simulink model "BMS_System_Arch"  (R2024a)
settings: Solver=VariableStepAuto  StartTime=0.0  StopTime=10.0  RelTol=1e-3
model workspace (MAT data in the model file):
  CANBusInterface = Simulink.Bus
  CANBusInterface.Alignment = -1
  CANBusInterface.PreserveElementDimensions = 0
  CANBusInterface.DataScope = 'Auto'
  ChargerInterface = Simulink.Bus
  ChargerInterface.Alignment = -1
  ChargerInterface.PreserveElementDimensions = 0
  ChargerInterface.DataScope = 'Auto'
  DataAcqBus = Simulink.Bus
  DataAcqBus.Alignment = -1
  DataAcqBus.PreserveElementDimensions = 0
  DataAcqBus.DataScope = 'Auto'
  DataCalcBus = Simulink.Bus
  DataCalcBus.Alignment = -1
  DataCalcBus.PreserveElementDimensions = 0
  DataCalcBus.DataScope = 'Auto'
  EstimationBusInterface = Simulink.Bus
  EstimationBusInterface.Alignment = -1
  EstimationBusInterface.PreserveElementDimensions = 0
  EstimationBusInterface.DataScope = 'Auto'
  HMIInterface = Simulink.Bus
  HMIInterface.Alignment = -1
  HMIInterface.PreserveElementDimensions = 0
  HMIInterface.DataScope = 'Auto'
  OperationControl = Simulink.Bus
  OperationControl.Alignment = -1
  OperationControl.PreserveElementDimensions = 0
  OperationControl.DataScope = 'Auto'
  SafetyInterface = Simulink.Bus
  SafetyInterface.Alignment = -1
  SafetyInterface.PreserveElementDimensions = 0
  SafetyInterface.DataScope = 'Auto'
  ThermalInterface = Simulink.Bus
  ThermalInterface.Alignment = -1
  ThermalInterface.PreserveElementDimensions = 0
  ThermalInterface.DataScope = 'Auto'
  UDSInterface = Simulink.Bus
  UDSInterface.Alignment = -1
  UDSInterface.PreserveElementDimensions = 0
  UDSInterface.DataScope = 'Auto'
settings Model: Creator=hirah  LastModifiedBy=hirah

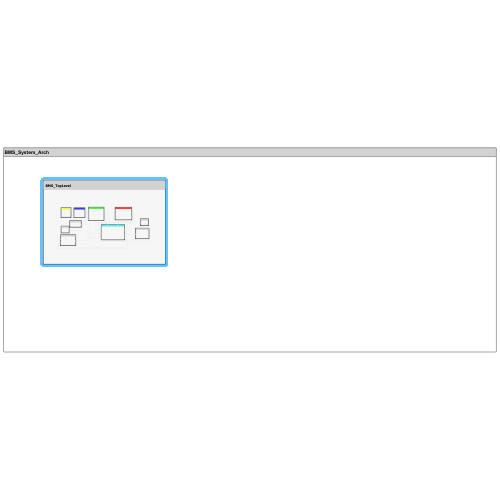
[thumbnail: Simulink's stored preview of the top-level diagram]
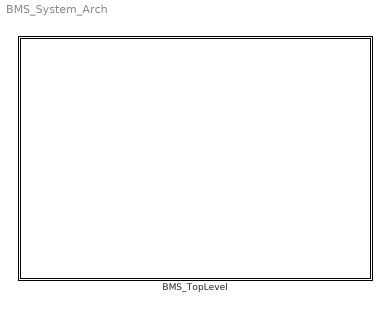
== system BMS_System_Arch ==
  BMS_TopLevel : Subsystem
      settings: PortSchema="{\"entries\":[{\"content\":{\"headerSize\":26,\"margin\":15,\"minimumSpacing\":25,\"sides\":[{\"content\":{},\"type\":\"ConnectorPlacement.EquallySpacedRectSide\",\"uuid\":\"0075fff4-e359-4ca3-82d3-62066e5371b3\"},{\"content\":{\"side\":\"RIGHT\"},\"type\":\"ConnectorPlacement.EquallySpacedRectSide\",\"uuid\":\"0762518f-8ff4-47a0-8585-614cecfccf10\"},{\"content\":{\"side\":\"TOP\"},\"type\":\"ConnectorPlacement.EquallySpacedRectSide\",\"uuid\":\"3af96ac8-a5e6-433b-be31-5dc09c2330cd\"}]},\"type\":\"ConnectorPlacement.EquallySpacedConnector\",\"uuid\":\"5c35ae06-51a0-47e4-81f3-25c096dd406a\"}],\"packageUris\":[\"http://schema.mathworks.com/mf0/Connector/R2020b\"],\"version\":\"1.0\"}"

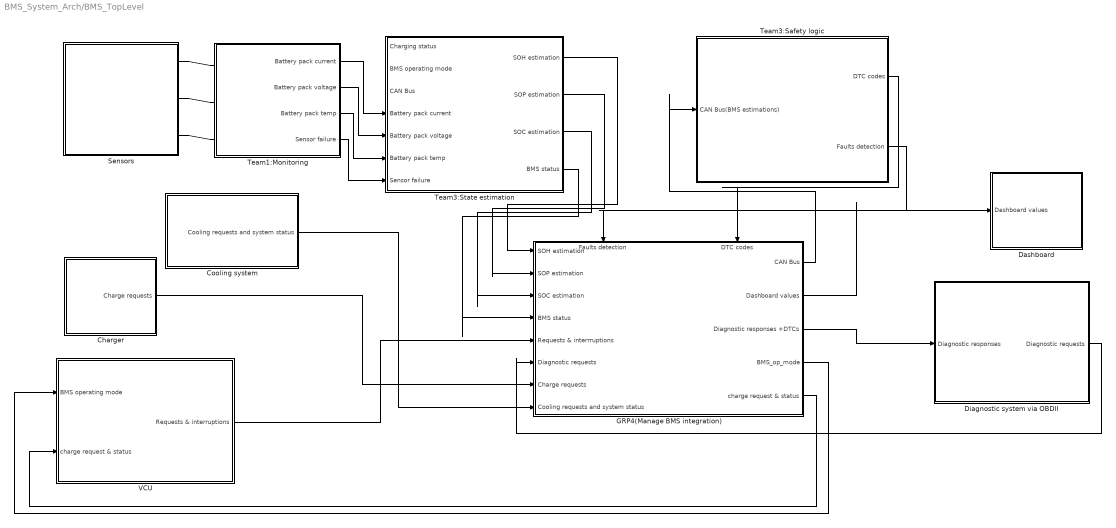
== system BMS_System_Arch/BMS_TopLevel ==
  Charger : Subsystem
      settings: PortSchema="{\"entries\":[{\"content\":{\"headerSize\":26,\"margin\":15,\"minimumSpacing\":25,\"sides\":[{\"content\":{},\"type\":\"ConnectorPlacement.EquallySpacedRectSide\",\"uuid\":\"cd2cdd02-8687-4a8c-9b6e-8ab5b03022cf\"},{\"content\":{\"connectorIds\":[\"Out1\"],\"side\":\"RIGHT\"},\"type\":\"ConnectorPlacement.EquallySpacedRectSide\",\"uuid\":\"c7d3337e-acaa-4958-9ee3-86e02c1b3b1e\"},{\"content\":{\"side\":\"TOP\"},\"type\":\"ConnectorPlacement.EquallySpacedRectSide\",\"uuid\":\"181ed1e6-99e4-4d5e-88b9-0d6c177ff349\"}]},\"type\":\"ConnectorPlacement.EquallySpacedConnector\",\"uuid\":\"35383a89-4be3-49fe-8681-3a2efe2b709c\"}],\"packageUris\":[\"http://schema.mathworks.com/mf0/Connector/R2020b\"],\"version\":\"1.0\"}"
  Cooling system : Subsystem
      settings: PortSchema="{\"entries\":[{\"content\":{\"headerSize\":26,\"margin\":15,\"minimumSpacing\":25,\"sides\":[{\"content\":{},\"type\":\"ConnectorPlacement.EquallySpacedRectSide\",\"uuid\":\"cd2cdd02-8687-4a8c-9b6e-8ab5b03022cf\"},{\"content\":{\"connectorIds\":[\"Out1\"],\"side\":\"RIGHT\"},\"type\":\"ConnectorPlacement.EquallySpacedRectSide\",\"uuid\":\"c7d3337e-acaa-4958-9ee3-86e02c1b3b1e\"},{\"content\":{\"side\":\"TOP\"},\"type\":\"ConnectorPlacement.EquallySpacedRectSide\",\"uuid\":\"181ed1e6-99e4-4d5e-88b9-0d6c177ff349\"}]},\"type\":\"ConnectorPlacement.EquallySpacedConnector\",\"uuid\":\"35383a89-4be3-49fe-8681-3a2efe2b709c\"}],\"packageUris\":[\"http://schema.mathworks.com/mf0/Connector/R2020b\"],\"version\":\"1.0\"}"
  Dashboard : Subsystem
      settings: PortSchema="{\"entries\":[{\"content\":{\"headerSize\":26,\"margin\":15,\"minimumSpacing\":25,\"sides\":[{\"content\":{\"connectorIds\":[\"In1\"]},\"type\":\"ConnectorPlacement.EquallySpacedRectSide\",\"uuid\":\"cd2cdd02-8687-4a8c-9b6e-8ab5b03022cf\"},{\"content\":{\"side\":\"RIGHT\"},\"type\":\"ConnectorPlacement.EquallySpacedRectSide\",\"uuid\":\"c7d3337e-acaa-4958-9ee3-86e02c1b3b1e\"},{\"content\":{\"side\":\"TOP\"},\"type\":\"ConnectorPlacement.EquallySpacedRectSide\",\"uuid\":\"181ed1e6-99e4-4d5e-88b9-0d6c177ff349\"}]},\"type\":\"ConnectorPlacement.EquallySpacedConnector\",\"uuid\":\"35383a89-4be3-49fe-8681-3a2efe2b709c\"}],\"packageUris\":[\"http://schema.mathworks.com/mf0/Connector/R2020b\"],\"version\":\"1.0\"}"
  Diagnostic system via OBDII : Subsystem
      settings: PortSchema="{\"entries\":[{\"content\":{\"headerSize\":26,\"margin\":15,\"minimumSpacing\":25,\"sides\":[{\"content\":{\"connectorIds\":[\"In1\"]},\"type\":\"ConnectorPlacement.EquallySpacedRectSide\",\"uuid\":\"cd2cdd02-8687-4a8c-9b6e-8ab5b03022cf\"},{\"content\":{\"connectorIds\":[\"Out1\"],\"side\":\"RIGHT\"},\"type\":\"ConnectorPlacement.EquallySpacedRectSide\",\"uuid\":\"c7d3337e-acaa-4958-9ee3-86e02c1b3b1e\"},{\"content\":{\"side\":\"TOP\"},\"type\":\"ConnectorPlacement.EquallySpacedRectSide\",\"uuid\":\"181ed1e6-99e4-4d5e-88b9-0d6c177ff349\"}]},\"type\":\"ConnectorPlacement.EquallySpacedConnector\",\"uuid\":\"35383a89-4be3-49fe-8681-3a2efe2b709c\"}],\"packageUris\":[\"http://schema.mathworks.com/mf0/Connector/R2020b\"],\"version\":\"1.0\"}"
  GRP4(Manage BMS integration) : Subsystem
      settings: PortSchema="{\"entries\":[{\"content\":{\"headerSize\":26,\"margin\":15,\"minimumSpacing\":25,\"sides\":[{\"content\":{\"connectorIds\":[\"In3\",\"In4\",\"In8\",\"In9\",\"In10\",\"In5\",\"In6\",\"In7\"]},\"type\":\"ConnectorPlacement.EquallySpacedRectSide\",\"uuid\":\"faff89d9-e9e4-4b6f-9f42-f9315910e0de\"},{\"content\":{\"connectorIds\":[\"Out1\",\"Out2\",\"Out3\",\"Out4\",\"Out5\"],\"side\":\"RIGHT\"},\"type\":\"ConnectorPlacement.EquallySpacedRectSide\",\"uuid\":\"9773bad6-87c4-4101-99c1-1d204d4e17cb\"},{\"content\":{\"connectorIds\":[\"In1\",\"In2\"],\"side\":\"TOP\"},\"type\":\"ConnectorPlacement.EquallySpacedRectSide\",\"uuid\":\"573ffa45-035d-496a-acbc-febfae678741\"}]},\"type\":\"ConnectorPlacement.EquallySpacedConnector\",\"uuid\":\"e66d261f-d4c2-4899-bd49-de4415fbe12f\"}],\"packageUris\":[\"http://schema.mathworks.com/mf0/Connector/R2020b\"],\"version\":\"1.0\"}"
  Sensors : Subsystem
      settings: PortSchema="{\"entries\":[{\"content\":{\"headerSize\":26,\"margin\":15,\"minimumSpacing\":25,\"sides\":[{\"content\":{},\"type\":\"ConnectorPlacement.EquallySpacedRectSide\",\"uuid\":\"faff89d9-e9e4-4b6f-9f42-f9315910e0de\"},{\"content\":{\"connectorIds\":[\"RConn1\",\"RConn2\",\"RConn3\"],\"side\":\"RIGHT\"},\"type\":\"ConnectorPlacement.EquallySpacedRectSide\",\"uuid\":\"9773bad6-87c4-4101-99c1-1d204d4e17cb\"},{\"content\":{\"side\":\"TOP\"},\"type\":\"ConnectorPlacement.EquallySpacedRectSide\",\"uuid\":\"573ffa45-035d-496a-acbc-febfae678741\"}]},\"type\":\"ConnectorPlacement.EquallySpacedConnector\",\"uuid\":\"e66d261f-d4c2-4899-bd49-de4415fbe12f\"}],\"packageUris\":[\"http://schema.mathworks.com/mf0/Connector/R2020b\"],\"version\":\"1.0\"}"
  Team1:Monitoring : Subsystem
      settings: PortSchema="{\"entries\":[{\"content\":{\"headerSize\":26,\"margin\":15,\"minimumSpacing\":25,\"sides\":[{\"content\":{\"connectorIds\":[\"LConn1\",\"LConn2\",\"LConn3\"]},\"type\":\"ConnectorPlacement.EquallySpacedRectSide\",\"uuid\":\"cd2cdd02-8687-4a8c-9b6e-8ab5b03022cf\"},{\"content\":{\"connectorIds\":[\"Out1\",\"Out2\",\"Out3\",\"Out4\"],\"side\":\"RIGHT\"},\"type\":\"ConnectorPlacement.EquallySpacedRectSide\",\"uuid\":\"c7d3337e-acaa-4958-9ee3-86e02c1b3b1e\"},{\"content\":{\"side\":\"TOP\"},\"type\":\"ConnectorPlacement.EquallySpacedRectSide\",\"uuid\":\"181ed1e6-99e4-4d5e-88b9-0d6c177ff349\"}]},\"type\":\"ConnectorPlacement.EquallySpacedConnector\",\"uuid\":\"35383a89-4be3-49fe-8681-3a2efe2b709c\"}],\"packageUris\":[\"http://schema.mathworks.com/mf0/Connector/R2020b\"],\"version\":\"1.0\"}"
  Team3:Safety logic : Subsystem
      settings: PortSchema="{\"entries\":[{\"content\":{\"headerSize\":26,\"margin\":15,\"minimumSpacing\":25,\"sides\":[{\"content\":{\"connectorIds\":[\"In1\"]},\"type\":\"ConnectorPlacement.EquallySpacedRectSide\",\"uuid\":\"cd2cdd02-8687-4a8c-9b6e-8ab5b03022cf\"},{\"content\":{\"connectorIds\":[\"Out1\",\"Out2\"],\"side\":\"RIGHT\"},\"type\":\"ConnectorPlacement.EquallySpacedRectSide\",\"uuid\":\"c7d3337e-acaa-4958-9ee3-86e02c1b3b1e\"},{\"content\":{\"side\":\"TOP\"},\"type\":\"ConnectorPlacement.EquallySpacedRectSide\",\"uuid\":\"181ed1e6-99e4-4d5e-88b9-0d6c177ff349\"}]},\"type\":\"ConnectorPlacement.EquallySpacedConnector\",\"uuid\":\"35383a89-4be3-49fe-8681-3a2efe2b709c\"}],\"packageUris\":[\"http://schema.mathworks.com/mf0/Connector/R2020b\"],\"version\":\"1.0\"}"
  Team3:State estimation : Subsystem
      settings: PortSchema="{\"entries\":[{\"content\":{\"headerSize\":26,\"margin\":15,\"minimumSpacing\":25,\"sides\":[{\"content\":{\"connectorIds\":[\"In1\",\"In2\",\"In3\",\"In4\",\"In5\",\"In6\",\"In7\"]},\"type\":\"ConnectorPlacement.EquallySpacedRectSide\",\"uuid\":\"faff89d9-e9e4-4b6f-9f42-f9315910e0de\"},{\"content\":{\"connectorIds\":[\"Out1\",\"Out2\",\"Out3\",\"Out4\"],\"side\":\"RIGHT\"},\"type\":\"ConnectorPlacement.EquallySpacedRectSide\",\"uuid\":\"9773bad6-87c4-4101-99c1-1d204d4e17cb\"},{\"content\":{\"side\":\"TOP\"},\"type\":\"ConnectorPlacement.EquallySpacedRectSide\",\"uuid\":\"573ffa45-035d-496a-acbc-febfae678741\"}]},\"type\":\"ConnectorPlacement.EquallySpacedConnector\",\"uuid\":\"e66d261f-d4c2-4899-bd49-de4415fbe12f\"}],\"packageUris\":[\"http://schema.mathworks.com/mf0/Connector/R2020b\"],\"version\":\"1.0\"}"
  VCU : Subsystem
      settings: PortSchema="{\"entries\":[{\"content\":{\"headerSize\":26,\"margin\":15,\"minimumSpacing\":25,\"sides\":[{\"content\":{\"connectorIds\":[\"In1\",\"In2\"]},\"type\":\"ConnectorPlacement.EquallySpacedRectSide\",\"uuid\":\"cd2cdd02-8687-4a8c-9b6e-8ab5b03022cf\"},{\"content\":{\"connectorIds\":[\"Out1\"],\"side\":\"RIGHT\"},\"type\":\"ConnectorPlacement.EquallySpacedRectSide\",\"uuid\":\"c7d3337e-acaa-4958-9ee3-86e02c1b3b1e\"},{\"content\":{\"side\":\"TOP\"},\"type\":\"ConnectorPlacement.EquallySpacedRectSide\",\"uuid\":\"181ed1e6-99e4-4d5e-88b9-0d6c177ff349\"}]},\"type\":\"ConnectorPlacement.EquallySpacedConnector\",\"uuid\":\"35383a89-4be3-49fe-8681-3a2efe2b709c\"}],\"packageUris\":[\"http://schema.mathworks.com/mf0/Connector/R2020b\"],\"version\":\"1.0\"}"
  wires:
  Team1:Monitoring/2(Battery pack voltage) -> Team3:State estimation/5(Battery pack voltage)
  Team1:Monitoring/1(Battery pack current) -> Team3:State estimation/4(Battery pack current)
  Team1:Monitoring/3(Battery pack temp) -> Team3:State estimation/6(Battery pack temp)
  Team1:Monitoring/4(Sensor failure) -> Team3:State estimation/7(Sensor failure)
  Team3:State estimation/1(SOH estimation) -> GRP4(Manage BMS integration)/3(SOH estimation)
  Team3:State estimation/2(SOP estimation) -> GRP4(Manage BMS integration)/4(SOP estimation)
  Team3:State estimation/3(SOC estimation) -> GRP4(Manage BMS integration)/8(SOC estimation)
  Team3:State estimation/4(BMS status) -> GRP4(Manage BMS integration)/9(BMS status)
  VCU/1(Requests & interruptions) -> GRP4(Manage BMS integration)/10(Requests & interrruptions)
  GRP4(Manage BMS integration)/1(CAN Bus) -> Team3:Safety logic/1(CAN Bus(BMS estimations))
  Team3:Safety logic/2(Faults detection) -> GRP4(Manage BMS integration)/1(Faults detection)
  Team3:Safety logic/1(DTC codes) -> GRP4(Manage BMS integration)/2(DTC codes)
  GRP4(Manage BMS integration)/4(BMS_op_mode) -> VCU/1(BMS operating mode)
  GRP4(Manage BMS integration)/3(Diagnostic responses +DTCs) -> Diagnostic system via OBDII/1(Diagnostic responses)
  Diagnostic system via OBDII/1(Diagnostic requests) -> GRP4(Manage BMS integration)/5(Diagnostic requests)
  GRP4(Manage BMS integration)/2(Dashboard values) -> Dashboard/1(Dashboard values)
  GRP4(Manage BMS integration)/5(charge request & status) -> VCU/2(charge request & status)
  Charger/1(Charge requests) -> GRP4(Manage BMS integration)/6(Charge requests)
  Cooling system/1(Cooling requests and system status) -> GRP4(Manage BMS integration)/7(Cooling requests and system status)
  connections:
  Sensors/RConn2 -- Team1:Monitoring/LConn2
  Sensors/RConn1 -- Team1:Monitoring/LConn1
  Sensors/RConn3 -- Team1:Monitoring/LConn3

== system BMS_System_Arch/BMS_TopLevel/Charger ==
  Bus Element Out1 : Outport  PortName=Charge requests

== system BMS_System_Arch/BMS_TopLevel/Cooling system ==
  Bus Element Out1 : Outport  PortName=Cooling requests and system status

== system BMS_System_Arch/BMS_TopLevel/Dashboard ==
  Bus Element In1 : Inport  PortName=Dashboard values

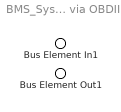
== system BMS_System_Arch/BMS_TopLevel/Diagnostic system via OBDII ==
  Bus Element In1 : Inport  PortName=Diagnostic responses
  Bus Element Out1 : Outport  PortName=Diagnostic requests

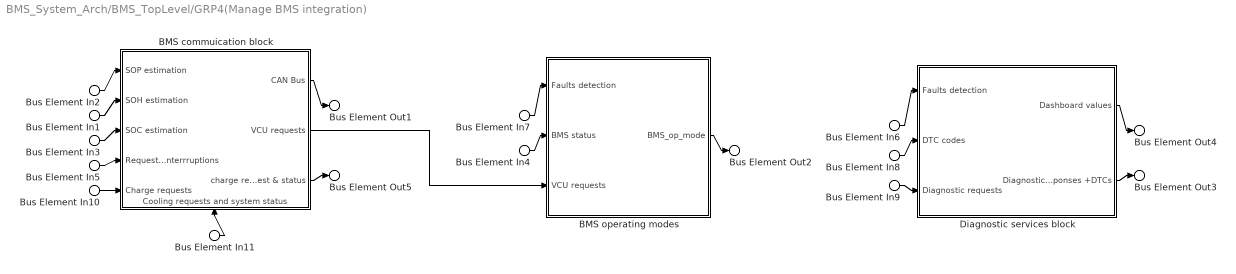
== system BMS_System_Arch/BMS_TopLevel/GRP4(Manage BMS integration) ==
  Bus Element In6 : Inport  PortName=Faults detection
  Bus Element In7 : Inport  PortName=Faults detection
  Bus Element In8 : Inport  Port=2  PortName=DTC codes
  Bus Element In1 : Inport  Port=3  PortName=SOH estimation
  Bus Element In2 : Inport  Port=4  PortName=SOP estimation
  Bus Element In9 : Inport  Port=5  PortName=Diagnostic requests
  Bus Element In10 : Inport  Port=6  PortName=Charge requests
  Bus Element In11 : Inport  Port=7  PortName=Cooling requests and system status
  Bus Element In3 : Inport  Port=8  PortName=SOC estimation
  Bus Element In4 : Inport  Port=9  PortName=BMS status
  Bus Element In5 : Inport  Port=10  PortName=Requests & interrruptions
  BMS commuication block : Subsystem
      settings: PortSchema="{\"entries\":[{\"content\":{\"headerSize\":26,\"margin\":15,\"minimumSpacing\":25,\"sides\":[{\"content\":{\"connectorIds\":[\"In2\",\"In3\",\"In4\",\"In5\",\"In6\"]},\"type\":\"ConnectorPlacement.EquallySpacedRectSide\",\"uuid\":\"04ec415f-b4bd-4017-972b-9e85e691a4fa\"},{\"content\":{\"connectorIds\":[\"Out1\",\"Out2\",\"Out3\"],\"side\":\"RIGHT\"},\"type\":\"ConnectorPlacement.EquallySpacedRectSide\",\"uuid\":\"35151384-2339-42ef-bb6e-a180feceabd8\"},{\"content\":{\"side\":\"TOP\"},\"type\":\"ConnectorPlacement.EquallySpacedRectSide\",\"uuid\":\"c25567f8-acdc-4fac-aea5-0e07a58d33ff\"},{\"content\":{\"connectorIds\":[\"In1\"],\"side\":\"BOTTOM\"},\"type\":\"ConnectorPlacement.EquallySpacedRectSide\",\"uuid\":\"03d92b78-152a-4a99-a80a-d3186856140b\"}]},\"type\":\"ConnectorPlacement.EquallySpacedConnector\",\"uuid\":\"6bdc95ed-225b-47c7-9236-872fc0620aae\"}],\"packageUris\":[\"http://schema.mathworks.com/mf0/Connector/R2020b\"],\"version\":\"1.0\"}"
  BMS operating modes : Subsystem
      settings: PortSchema="{\"entries\":[{\"content\":{\"headerSize\":26,\"margin\":15,\"minimumSpacing\":25,\"sides\":[{\"content\":{\"connectorIds\":[\"In1\",\"In2\",\"In3\"]},\"type\":\"ConnectorPlacement.EquallySpacedRectSide\",\"uuid\":\"faff89d9-e9e4-4b6f-9f42-f9315910e0de\"},{\"content\":{\"connectorIds\":[\"Out1\"],\"side\":\"RIGHT\"},\"type\":\"ConnectorPlacement.EquallySpacedRectSide\",\"uuid\":\"9773bad6-87c4-4101-99c1-1d204d4e17cb\"},{\"content\":{\"side\":\"TOP\"},\"type\":\"ConnectorPlacement.EquallySpacedRectSide\",\"uuid\":\"573ffa45-035d-496a-acbc-febfae678741\"}]},\"type\":\"ConnectorPlacement.EquallySpacedConnector\",\"uuid\":\"e66d261f-d4c2-4899-bd49-de4415fbe12f\"}],\"packageUris\":[\"http://schema.mathworks.com/mf0/Connector/R2020b\"],\"version\":\"1.0\"}"
  Diagnostic services block : Subsystem
      settings: PortSchema="{\"entries\":[{\"content\":{\"headerSize\":26,\"margin\":15,\"minimumSpacing\":25,\"sides\":[{\"content\":{\"connectorIds\":[\"In1\",\"In2\",\"In3\"]},\"type\":\"ConnectorPlacement.EquallySpacedRectSide\",\"uuid\":\"04ec415f-b4bd-4017-972b-9e85e691a4fa\"},{\"content\":{\"connectorIds\":[\"Out1\",\"Out2\"],\"side\":\"RIGHT\"},\"type\":\"ConnectorPlacement.EquallySpacedRectSide\",\"uuid\":\"35151384-2339-42ef-bb6e-a180feceabd8\"},{\"content\":{\"side\":\"TOP\"},\"type\":\"ConnectorPlacement.EquallySpacedRectSide\",\"uuid\":\"c25567f8-acdc-4fac-aea5-0e07a58d33ff\"}]},\"type\":\"ConnectorPlacement.EquallySpacedConnector\",\"uuid\":\"6bdc95ed-225b-47c7-9236-872fc0620aae\"}],\"packageUris\":[\"http://schema.mathworks.com/mf0/Connector/R2020b\"],\"version\":\"1.0\"}"
  Bus Element Out1 : Outport  PortName=CAN Bus
  Bus Element Out4 : Outport  Port=2  PortName=Dashboard values
  Bus Element Out3 : Outport  Port=3  PortName=Diagnostic responses +DTCs
  Bus Element Out2 : Outport  Port=4  PortName=BMS_op_mode
  Bus Element Out5 : Outport  Port=5  PortName=charge request & status
  wires:
  Diagnostic services block/1(Dashboard values) -> Bus Element Out4/1
  Diagnostic services block/2(Diagnostic responses +DTCs) -> Bus Element Out3/1
  BMS commuication block/1(CAN Bus) -> Bus Element Out1/1
  Bus Element In8/1 -> Diagnostic services block/2(DTC codes)
  Bus Element In6/1 -> Diagnostic services block/1(Faults detection)
  Bus Element In1/1 -> BMS commuication block/3(SOH estimation)
  Bus Element In2/1 -> BMS commuication block/2(SOP estimation)
  Bus Element In3/1 -> BMS commuication block/4(SOC estimation)
  Bus Element In4/1 -> BMS operating modes/2(BMS status)
  Bus Element In5/1 -> BMS commuication block/5(Requests & interrruptions)
  BMS commuication block/2(VCU requests) -> BMS operating modes/3(VCU requests)
  Bus Element In9/1 -> Diagnostic services block/3(Diagnostic requests)
  Bus Element In10/1 -> BMS commuication block/6(Charge requests)
  Bus Element In11/1 -> BMS commuication block/1(Cooling requests and system status)
  BMS operating modes/1(BMS_op_mode) -> Bus Element Out2/1
  BMS commuication block/3(charge request & status) -> Bus Element Out5/1
  Bus Element In7/1 -> BMS operating modes/1(Faults detection)

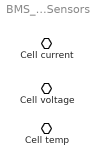
== system BMS_System_Arch/BMS_TopLevel/Sensors ==
  Cell current : PMIOPort  Side=Right
  Cell voltage : PMIOPort  Port=2  Side=Right
  Cell temp : PMIOPort  Port=3  Side=Right

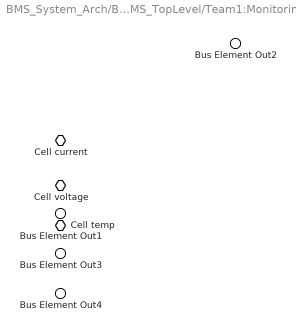
== system BMS_System_Arch/BMS_TopLevel/Team1:Monitoring ==
  Cell current : PMIOPort  Side=Left  ConnectionType=Connection: foundation.electrical.eight_phase
  Cell voltage : PMIOPort  Port=2  Side=Left
  Cell temp : PMIOPort  Port=3  Side=Left
  Bus Element Out2 : Outport  PortName=Battery pack current
  Bus Element Out1 : Outport  Port=2  PortName=Battery pack voltage
  Bus Element Out3 : Outport  Port=3  PortName=Battery pack temp
  Bus Element Out4 : Outport  Port=4  PortName=Sensor failure

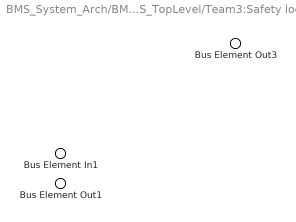
== system BMS_System_Arch/BMS_TopLevel/Team3:Safety logic ==
  Bus Element In1 : Inport  PortName=CAN Bus(BMS estimations)
  Bus Element Out3 : Outport  PortName=DTC codes
  Bus Element Out1 : Outport  Port=2  PortName=Faults detection

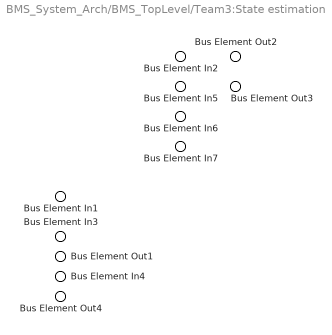
== system BMS_System_Arch/BMS_TopLevel/Team3:State estimation ==
  Bus Element In7 : Inport  PortName=Charging status
  Bus Element In6 : Inport  Port=2  PortName=BMS operating mode
  Bus Element In5 : Inport  Port=3  PortName=CAN Bus
  Bus Element In2 : Inport  Port=4  PortName=Battery pack current
  Bus Element In1 : Inport  Port=5  PortName=Battery pack voltage
  Bus Element In3 : Inport  Port=6  PortName=Battery pack temp
  Bus Element In4 : Inport  Port=7  PortName=Sensor failure
  Bus Element Out2 : Outport  PortName=SOH estimation
  Bus Element Out3 : Outport  Port=2  PortName=SOP estimation
  Bus Element Out1 : Outport  Port=3  PortName=SOC estimation
  Bus Element Out4 : Outport  Port=4  PortName=BMS status

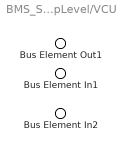
== system BMS_System_Arch/BMS_TopLevel/VCU ==
  Bus Element In1 : Inport  PortName=BMS operating mode
  Bus Element In2 : Inport  Port=2  PortName=charge request & status
  Bus Element Out1 : Outport  PortName=Requests & interruptions

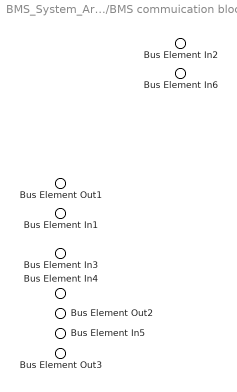
== system BMS_System_Arch/BMS_TopLevel/GRP4(Manage BMS integration)/BMS commuication block ==
  Bus Element In6 : Inport  PortName=Cooling requests and system status
  Bus Element In2 : Inport  Port=2  PortName=SOP estimation
  Bus Element In1 : Inport  Port=3  PortName=SOH estimation
  Bus Element In3 : Inport  Port=4  PortName=SOC estimation
  Bus Element In4 : Inport  Port=5  PortName=Requests & interrruptions
  Bus Element In5 : Inport  Port=6  PortName=Charge requests
  Bus Element Out1 : Outport  PortName=CAN Bus
  Bus Element Out2 : Outport  Port=2  PortName=VCU requests
  Bus Element Out3 : Outport  Port=3  PortName=charge request & status

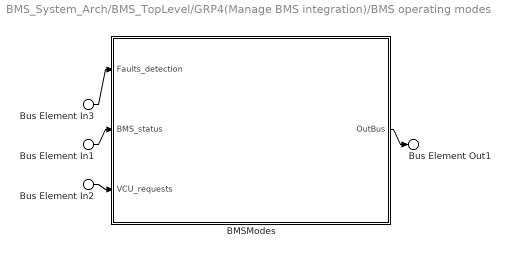
== system BMS_System_Arch/BMS_TopLevel/GRP4(Manage BMS integration)/BMS operating modes ==
  Bus Element In3 : Inport  PortName=Faults detection
  Bus Element In1 : Inport  Port=2  PortName=BMS status
  Bus Element In2 : Inport  Port=3  PortName=VCU requests
  BMSModes : Stateflow chart  TreatAsAtomicUnit=on
      settings: PortSchema="{\"entries\":[{\"content\":{\"headerSize\":26,\"margin\":15,\"minimumSpacing\":25,\"sides\":[{\"content\":{\"connectorIds\":[\"In1\",\"In2\",\"In3\"]},\"type\":\"ConnectorPlacement.EquallySpacedRectSide\",\"uuid\":\"04ec415f-b4bd-4017-972b-9e85e691a4fa\"},{\"content\":{\"connectorIds\":[\"Out1\"],\"side\":\"RIGHT\"},\"type\":\"ConnectorPlacement.EquallySpacedRectSide\",\"uuid\":\"35151384-2339-42ef-bb6e-a180feceabd8\"},{\"content\":{\"side\":\"TOP\"},\"type\":\"ConnectorPlacement.EquallySpacedRectSide\",\"uuid\":\"c25567f8-acdc-4fac-aea5-0e07a58d33ff\"}]},\"type\":\"ConnectorPlacement.EquallySpacedConnector\",\"uuid\":\"6bdc95ed-225b-47c7-9236-872fc0620aae\"}],\"packageUris\":[\"http://schema.mathworks.com/mf0/Connector/R2020b\"],\"version\":\"1.0\"}"
  Bus Element Out1 : Outport  PortName=BMS_op_mode
  wires:
  Bus Element In1/1 -> BMSModes/2(BMS_status)
  Bus Element In2/1 -> BMSModes/3(VCU_requests)
  Bus Element In3/1 -> BMSModes/1(Faults_detection)
  BMSModes/1(OutBus) -> Bus Element Out1/1

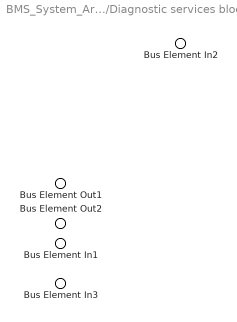
== system BMS_System_Arch/BMS_TopLevel/GRP4(Manage BMS integration)/Diagnostic services block ==
  Bus Element In2 : Inport  PortName=Faults detection
  Bus Element In1 : Inport  Port=2  PortName=DTC codes
  Bus Element In3 : Inport  Port=3  PortName=Diagnostic requests
  Bus Element Out1 : Outport  PortName=Dashboard values
  Bus Element Out2 : Outport  Port=2  PortName=Diagnostic responses +DTCs

== stateflow chart BMS_System_Arch/BMS_TopLevel/GRP4(Manage BMS integration)/BMS operating modes/BMSModes ==
  state Init
    en:
    BMS_op_mode= BMSModes.BMS_init;
  state Normal
    en:
    BMS_op_mode= BMSModes.BMS_normal;
  state Standby
    en:
    BMS_op_mode= BMSModes.BMS_standby;
  state Charging
    en:
    BMS_op_mode= BMSModes.BMS_charging;
  state Shutdown
    en:
    BMS_op_mode= BMSModes.BMS_shutdown;
  state Fault
    en:
    BMS_op_mode= BMSModes.BMS_fault;
  Charging -> Standby [order 2] : [VCU_request==ChargingComplete]
  Standby -> Charging [order 2] : [VCU_request==ChargeBegin]
  (default) -> Standby
  Standby -> Init [order 1] : [VCU_requests == BMSModes.BMS_init]
  Init -> Normal [order 1] : [VCU_requests == BMSModes.BMS_normal]
  Init -> Shutdown [order 2] : [VCU_request==PowerOFF]
  Fault -> Standby [order 2] : [VCU_request==FaultCleared]
  Shutdown -> Standby : [VCU_request==wakeUp]
  Normal -> Fault : [VCU_request==CriticalFault]
  Charging -> Fault [order 1] : [VCU_request==ChargingFault]
  Fault -> Shutdown [order 1] : [VCU_request==CriticalFailure]
  data: Faults_detection input; BMS_status input; VCU_requests input; OutBus output
